simulink model "PIDpenduloInvertido"  (R2020b)
settings: Solver=ode4  StartTime=0.0  StopTime=180  FixedStep=0.05  RelTol=1e-3
model workspace (MAT data in the model file):
  Ts = 0.05
  kdt = -30134.5435307
  kit = -43476.4735237
  kpt = -72391.8140113
  ref = 0.0349065850399
values from neighbouring files (symbols this model uses):
  g = 9.81    [PIDMiplanta.m]    (also in PID_Pendulo.m)
  l = 1.5    [PIDMiplanta.m]    (also in PID_Pendulo.m = 6.096)
  M = 583.756    [PIDMiplanta.m]    (also in PID_Pendulo.m)
  m = 116.7512    [PIDMiplanta.m]    (also in PID_Pendulo.m)
libraries: vrlib x3, pid_lib x1, dspsrcs4 x1, commchan3 x1
settings Model: OrderedModelArguments=off  Creator=Matias  LastModifiedBy=Matias

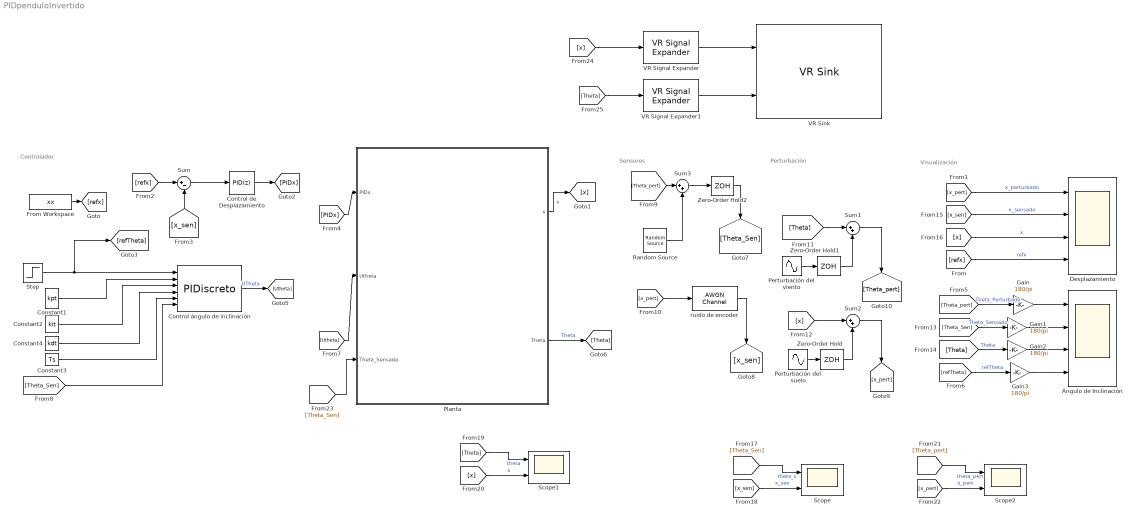
== system PIDpenduloInvertido ==
  note: Perturbación
  note: Sensores
  note: Visualización
  note: Controlador
  Constant1 : Constant  Value=kpt  SampleTime=-1
  Constant2 : Constant  Value=kit  SampleTime=-1
  Constant3 : Constant  Value=Ts  SampleTime=-1
  Constant4 : Constant  Value=kdt  SampleTime=-1
  Control de Desplazamiento : pid_lib/PID Controller  Controller=PID  Form=Parallel  TimeDomain=Discrete-time  UseExternalTs=off  SampleTime=-1  IntegratorMethod=Forward Euler  FilterMethod=Forward Euler  ControllerParametersSource=internal  P=0.032482967957332  I=0.00227243206651007  D=0.110339112095264  UseFilter=on  N=2.80224211839692  TunerSelectOption=Transfer Function Based (PID Tuner App)  InitialConditionSource=internal  InitialConditionForIntegrator=0  InitialConditionForFilter=0  DifferentiatorICPrevScaledInput=0  ExternalReset=none  TrackingMode=off  Kt=1  LimitOutput=off  SatLimitsSource=internal  UpperSaturationLimit=inf  LowerSaturationLimit=-inf  LinearizeAsGain=off  AntiWindupMode=none  Kb=1  POutMin=[]  POutMax=[]  IOutMin=[]  IOutMax=[]  DOutMin=[]  DOutMax=[]  NOutMin=[]  NOutMax=[]  SumOutMin=[]  SumOutMax=[]  SaturationOutMin=[]  SaturationOutMax=[]  PParamMin=[]  PParamMax=[]  IParamMin=[]  IParamMax=[]  DParamMin=[]  DParamMax=[]  NParamMin=[]  NParamMax=[]  KbParamMin=[]  KbParamMax=[]  KtParamMin=[]  KtParamMax=[]  KbOutMin=[]  KbOutMax=[]  KtOutMin=[]  KtOutMax=[]  IntegratorOutMin=[]  IntegratorOutMax=[]  FilterOutMin=[]  FilterOutMax=[]  SumI1OutMin=[]  SumI1OutMax=[]  SumI2OutMin=[]  SumI2OutMax=[]  SumI3OutMin=[]  SumI3OutMax=[]  SumI4OutMin=[]  SumI4OutMax=[]  SumDOutMin=[]  SumDOutMax=[]  DifferentiatorOutMin=[]  DifferentiatorOutMax=[]  FilterDiffOutCoefMin=[]  FilterDiffOutCoefMax=[]  ReciprocalOutMin=[]  ReciprocalOutMax=[]  SumDenOutMin=[]  SumDenOutMax=[]  SumNumOutMin=[]  SumNumOutMax=[]  DivideOutMin=[]  DivideOutMax=[]  UdiffTsProdOutMin=[]  UdiffTsProdOutMax=[]  NTsProdOutMin=[]  NTsProdOutMax=[]  UintegralTsProdOutMin=[]  UintegralTsProdOutMax=[]  UngainTsProdOutMin=[]  UngainTsProdOutMax=[]  IntegratorContinuousStateAttributes=''  IntegratorStateMustResolveToSignalObject=off  IntegratorRTWStateStorageClass=Auto  FilterContinuousStateAttributes=''  FilterStateMustResolveToSignalObject=off  FilterRTWStateStorageClass=Auto  ParallelPVariant=InternalParameters  IdealPVariant=Disabled  IVariant=InternalParameters  DVariant=InternalParameters  IntegratorVariant=Discrete  SatVariant=Disabled  AWVariant=Passthrough  PCopyVariant=Disabled  TRVariant=Disabled  FdbkBlocksVariant=Forward  IdealPFdbkVariant=Disabled  SatFdbkVariant=Disabled  DerivativeFilterVariant=ForwardEulerFilter  NVariant=InternalParameters  NCopyVariant=Disabled  FilterICVariant=InternalICsFilter  IntegratorICVariant=InternalICs  ExternalResetVariant=Disabled  TRSumVariant=Passthrough  SumFdbkVariant=Disabled  SumVariant=Sum_PID  TsampFilterVariant=InternalTs  TsampNgainVariant=Passthrough  TsampIntegralVariant=Passthrough  ExternalSaturationOutDataTypeStr=Inherit: Same as second input
  Control ángulo de inclinación : S-Function  FunctionName=PIDiscreto  SFunctionDeploymentMode=off  EnableBusSupport=off
  Desplazamiento : Scope  NumInputPorts=4
  From Workspace : FromWorkspace  VariableName=xx
  Gain{,1..3} (4 alike) : Gain  Gain=180/pi
  Perturbación del suelo : Sin  Amplitude=0.001  Frequency=0.05  SampleTime=0
  Perturbación del viento : Sin  Amplitude=0.01  Frequency=0.07  SampleTime=0
  Planta : Subsystem
  Random Source : dspsrcs4/Random Source  SrcType=Gaussian  NormMethod=Ziggurat  CltLength=12  MinVal=0  MaxVal=1  MeanVal=0  VarVal=var_Theta  RepMode=Not repeatable  rawSeed=1  IsInherit=off  SampMode=Discrete  SampTime=-1  SampFrame=1  DataType=Double  OutComplex=Real  OutputFrames=off
  Scope : Scope  NumInputPorts=2
  Scope1 : Scope  NumInputPorts=2
  Scope2 : Scope  NumInputPorts=2
  Step : Step  After=0*pi/180  SampleTime=0
  Sum : Sum  Inputs=|+-
  Sum1 : Sum  Inputs=|++
  Sum2 : Sum  Inputs=|++
  Sum3 : Sum  Inputs=|++
  VR Signal Expander : vrlib/VR Signal Expander  outwidth=3  outidx=1
  VR Signal Expander1 : vrlib/VR Signal Expander  outwidth=4  outidx=4
  VR Sink : vrlib/VR Sink  InstantiateOnLoad=on  SampleTime=0.05  ViewEnable=on  RemoteChange=off  RemoteView=off  FieldsWritten=Carro.translation.3.1.1.double#ArticulacionPendulo.rotation.4.1.1.double  WorldFileName=penduloCarro.wrl  AutoView=off  VideoDimensions=[]  AllowVariableSize=off
  Zero-Order Hold : ZeroOrderHold  SampleTime=-1
  Zero-Order Hold1 : ZeroOrderHold  SampleTime=-1
  Zero-Order Hold2 : ZeroOrderHold  SampleTime=-1
  ruido de encoder : commchan3/AWGN Channel  InputProcessing=Columns as channels (frame based)  seed=67  noiseMode="Signal to noise ratio  (SNR)"  EbNodB=10  EsNodB=10  SNRdB=SNR_x  bitsPerSym=1  Ps=1  Tsym=1  variance=1
  Ángulo de Inclinación : Scope  NumInputPorts=4
  wires:
  Planta/1(x) -> [x]  "x"
  [refx] -> Desplazamiento/4  "refx"
  [x_pert] -> Desplazamiento/1  "x_perturbado"
  [PIDx] -> Planta/1(PIDx)
  [refTheta] -> Gain3/1  "refTheta"
  [Utheta] -> Planta/2(Utheta)
  Planta/2(Theta) -> [Theta]  "Theta"
  Constant4/1 -> Control ángulo de inclinación/4
  Constant1/1 -> Control ángulo de inclinación/2
  Step/1 -> [refTheta], Control ángulo de inclinación/1
  Control ángulo de inclinación/1 -> [Utheta]  "UTheta"
  [x_sen] -> Sum/2
  Constant2/1 -> Control ángulo de inclinación/3
  Constant3/1 -> Control ángulo de inclinación/5
  [Theta_Sen] -> Control ángulo de inclinación/6
  [refx] -> Sum/1
  Control de Desplazamiento/1 -> [PIDx]
  Sum/1 -> Control de Desplazamiento/1
  Zero-Order Hold2/1 -> [Theta_Sen]
  ruido de encoder/1 -> [x_sen]
  [Theta] -> Sum1/1
  [x] -> Sum2/1
  Sum2/1 -> [x_pert]
  Sum1/1 -> [Theta_pert]
  [Theta_pert] -> Gain/1  "Theta_Perturbado"
  [Theta_Sen] -> Gain1/1  "Theta_Sensado"
  [Theta] -> Gain2/1  "Theta"
  [x_sen] -> Desplazamiento/2  "x_sensado"
  [x] -> Desplazamiento/3  "x"
  [x_pert] -> ruido de encoder/1
  [Theta_Sen] -> Scope/1  "theta_s"
  [x_sen] -> Scope/2  "x_sen"
  [Theta] -> Scope1/1  "theta"
  [x] -> Scope1/2  "x"
  [Theta_pert] -> Scope2/1  "theta_pert"
  [x_pert] -> Scope2/2  "x_pert"
  Perturbación del suelo/1 -> Zero-Order Hold/1
  Zero-Order Hold/1 -> Sum2/2
  Perturbación del viento/1 -> Zero-Order Hold1/1
  Zero-Order Hold1/1 -> Sum1/2
  From Workspace/1 -> [refx]
  [Theta_pert] -> Sum3/1
  Random Source/1 -> Sum3/2
  Sum3/1 -> Zero-Order Hold2/1
  [Theta_Sen] -> Planta/3(Theta_Sensada)
  VR Signal Expander/1 -> VR Sink/1
  VR Signal Expander1/1 -> VR Sink/2
  [x] -> VR Signal Expander/1
  [Theta] -> VR Signal Expander1/1
  Gain/1 -> Ángulo de Inclinación/1
  Gain1/1 -> Ángulo de Inclinación/2
  Gain2/1 -> Ángulo de Inclinación/3
  Gain3/1 -> Ángulo de Inclinación/4

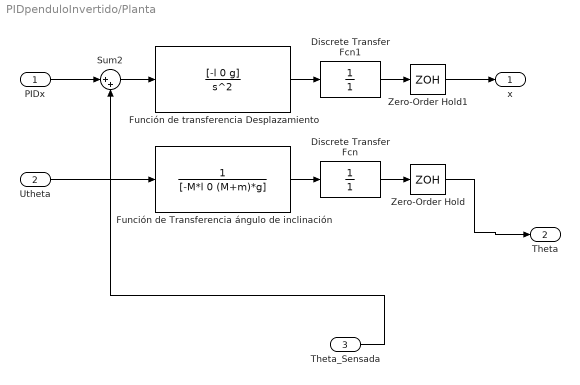
== system PIDpenduloInvertido/Planta ==
  PIDx : Inport
  Utheta : Inport  Port=2
  Theta_Sensada : Inport  Port=3
  Discrete Transfer Fcn : DiscreteTransferFcn  Denominator=[1]
  Discrete Transfer Fcn1 : DiscreteTransferFcn  Denominator=[1]
  Función de Transferencia ángulo de inclinación : TransferFcn  Denominator=[-M*l 0 (M+m)*g]
  Función de transferencia Desplazamiento : TransferFcn  Numerator=[-l 0 g]  Denominator=[1 0 0]
  Sum2 : Sum  Inputs=|++
  Zero-Order Hold : ZeroOrderHold  SampleTime=-1
  Zero-Order Hold1 : ZeroOrderHold  SampleTime=-1
  x : Outport
  Theta : Outport  Port=2
  wires:
  Utheta/1 -> Función de Transferencia ángulo de inclinación/1
  Sum2/1 -> Función de transferencia Desplazamiento/1
  Zero-Order Hold/1 -> Theta/1
  Función de Transferencia ángulo de inclinación/1 -> Discrete Transfer Fcn/1
  Discrete Transfer Fcn1/1 -> Zero-Order Hold1/1
  Zero-Order Hold1/1 -> x/1
  Discrete Transfer Fcn/1 -> Zero-Order Hold/1
  Función de transferencia Desplazamiento/1 -> Discrete Transfer Fcn1/1
  PIDx/1 -> Sum2/1
  Theta_Sensada/1 -> Sum2/2
